simulink model "sim_three_hop"  (R2020b)
settings: Solver=VariableStepAuto  StartTime=0.0  StopTime=1000  RelTol=1e-3  EnableMultiTasking=on
values from neighbouring files (symbols this model uses):
  sim_vars = [ 0, 0.9                8, 1,               8, 1,               8, 1,               inf, inf, inf                rand(1,1)*100000 ]    [main.m]
undefined symbols (not defined in the file or in its folder): m, n
settings Model: SimulationMode=accelerator  Creator=The MathWorks, Inc.  LastModifiedBy=ssmos
settings DataIOCC: LimitDataPoints=on  SaveOperatingPoint=on  SaveFormat=StructureWithTime
settings OptimizationCC: LifeSpan=inf
settings DebuggingCC: AllowSymbolicDim=off  SFUnexpectedBacktrackingDiag=warning  SFNoUnconditionalDefaultTransitionDiag=warning  SFExecutionAtInitializationDiag=none  ArithmeticOperatorsInVariantConditions=warning
settings ModelReferenceCC: PropagateSignalLabelsOutOfModel=off
settings SFSimCC: SimUseLocalCustomCode=off  CustomCodeUndefinedFunction=UseInterfaceOnly
settings RTWCC: RTWUseLocalCustomCode=off
settings CodeAppCC: StateflowObjectComments=on
settings GRTTargetCC: TargetLangStandard=C89/C90 (ANSI)
settings ConfigComp: CovMetricSettings=dw  CovSaveCumulativeToWorkspaceVar=on  CovSaveSingleToWorkspaceVar=on  CovExternalEMLEnable=off  CovSFcnEnable=off

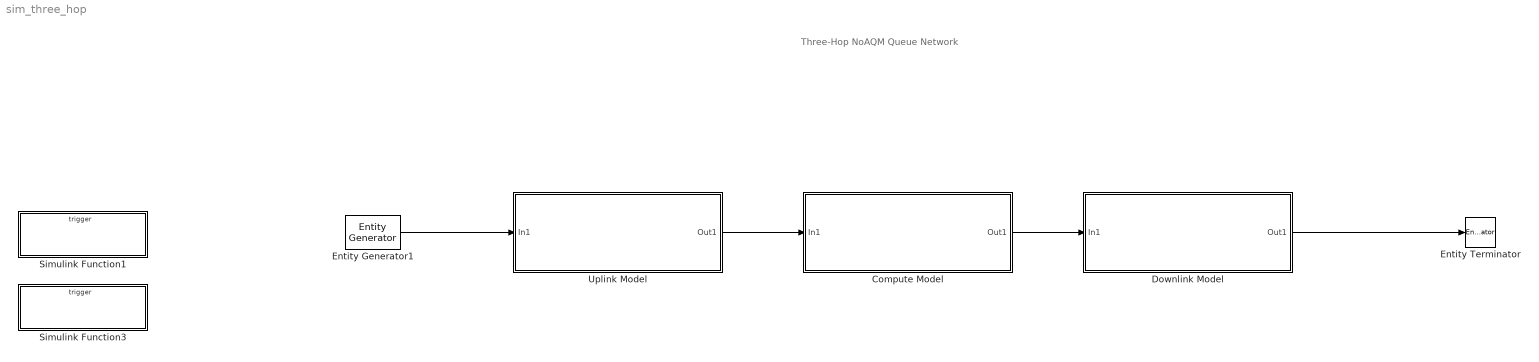
== system sim_three_hop ==
  note: Three-Hop NoAQM Queue Network
  Compute Model : Subsystem
  Downlink Model : Subsystem
  Entity Generator1 : EntityGenerator  OutputPortMessageModes=m  TimeSource=MATLAB action  IntergenerationTimeAction=dt = getArrivalTime(sim_vars(1),sim_vars(2),sim_vars(12));  GenerateAction=|  AttributeName=starttime|queuen_uplink_bu|servern_uplink_bu|queuen_compute_bu|servern_compute_bu|queuen_downlink_bu|servern_downlink_bu|queuen_compute_bc|servern_compute_bc|queuen_downlink_bc|servern_downlink_bc|queuen_downlink_bd|servern_downlink_bd|queuetime_uplink|servicetime_uplink|queuetime_compute|servicetime_compute|queuetime_downlink|servicetime_downlink|endtime  AttributeInitialValue=inf|-1|-1|-1|-1|-1|-1|-1|-1|-1|-1|-1|-1|inf|inf|inf|inf|inf|inf|inf  EntityType=Structured  EntityTypeName=Entity
      | entity.starttime = getCurrentTime();
      | 
      | entity.queuen_uplink_bu = getQueueNUplink();
      | entity.servern_uplink_bu = getServerNUplink();
      | 
      | entity.queuen_compute_bu = getQueueNCompute();
      | entity.servern_compute_bu = getServerNCompute();
      | 
      | entity.queuen_downlink_bu = getQueueNDownlink();
      | entity.servern_downlink_bu = getServerNDownlink();
      | 
      | %[nd,ne,np] = saveCrossNUplink();
      | %entity.crossn_uplink = nd-ne-np;
  Entity Terminator : EntityTerminator  InputPortMessageModes=m  EntryAction=|
      | entity.endtime = getCurrentTime();
      | 
      | saveAttributes([entity.starttime;               ...
      |                 entity.queuen_uplink_bu;        ...
      |                 entity.servern_uplink_bu;       ...
      |                 entity.queuen_compute_bu;       ...
      |                 entity.servern_compute_bu;      ...
      |                 entity.queuen_downlink_bu;      ...
      |                 entity.servern_downlink_bu;     ...
      |                 entity.queuen_compute_bc;       ...
      |                 entity.servern_compute_bc;      ...
      |                 entity.queuen_downlink_bc;      ...
      |                 entity.servern_downlink_bc;     ...
      |                 entity.queuen_downlink_bd;      ...
      |                 entity.servern_downlink_bd;     ...
      |                 entity.queuetime_uplink;        ...
      |                 entity.servicetime_uplink;      ...
      |                 entity.queuetime_compute;       ...
      |                 entity.servicetime_compute;     ...
      |                 entity.queuetime_downlink;      ...
      |                 entity.servicetime_downlink;    ...
      |                 entity.endtime;                 ...
      |                 entitySys.id]);
  Simulink Function1 : Subsystem  TreatAsAtomicUnit=on
  Simulink Function3 : Subsystem  TreatAsAtomicUnit=on
  Uplink Model : Subsystem
  wires:
  Entity Generator1/1 -> Uplink Model/1(In1)
  Uplink Model/1(Out1) -> Compute Model/1(In1)
  Downlink Model/1(Out1) -> Entity Terminator/1
  Compute Model/1(Out1) -> Downlink Model/1(In1)

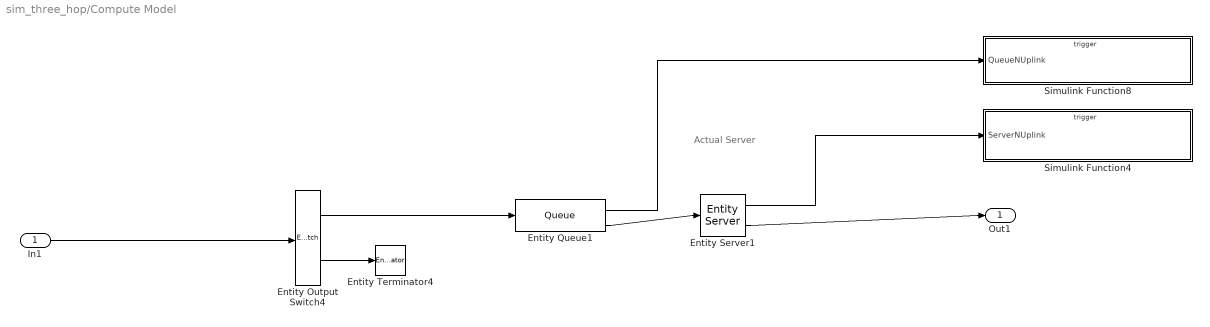
== system sim_three_hop/Compute Model ==
  note: Actual Server
  In1 : Inport
  Entity Output Switch4 : EntityOutputSwitch  InputPortMessageModes=m  OutputPortMessageModes=m,m  SwitchAttributeName=drop_at_source
  Entity Queue1 : Queue  InputPortMessageModes=m  OutputPortMessageModes=n,m  Capacity=sim_vars(10)  NumberEntitiesInBlock=on
      settings: OutputPortMap=o1,o5
  Entity Server1 : EntityServer  InputPortMessageModes=m  OutputPortMessageModes=n,m  Capacity=1  ServiceTimeSource=MATLAB action  ServiceTimeAction=dt = getServiceTimeCompute(sim_vars(5),sim_vars(6),sim_vars(12));  EntryAction=|  ServiceCompleteAction=|  NumberEntitiesInBlock=on
      EntryAction=|
      | % record packet's queue timestamp
      | entity.queuetime_compute = getCurrentTime();
      ServiceCompleteAction=|
      | % record service timestamp
      | entity.servicetime_compute = getCurrentTime();
      | 
      | % record network state in front
      | entity.queuen_downlink_bd = getQueueNDownlink();
      | entity.servern_downlink_bd = getServerNDownlink();
      settings: OutputPortMap=o1,o9
  Entity Terminator4 : EntityTerminator  InputPortMessageModes=m  EntryAction=|
      | saveAttributes([entity.starttime;               ...
      |                 entity.queuen_uplink_bu;        ...
      |                 entity.servern_uplink_bu;       ...
      |                 entity.queuen_compute_bu;       ...
      |                 entity.servern_compute_bu;      ...
      |                 entity.queuen_downlink_bu;      ...
      |                 entity.servern_downlink_bu;     ...
      |                 entity.queuen_compute_bc;       ...
      |                 entity.servern_compute_bc;      ...
      |                 entity.queuen_downlink_bc;      ...
      |                 entity.servern_downlink_bc;     ...
      |                 entity.queuen_downlink_bd;      ...
      |                 entity.servern_downlink_bd;     ...
      |                 entity.queuetime_uplink;        ...
      |                 entity.servicetime_uplink;      ...
      |                 entity.queuetime_compute;       ...
      |                 entity.servicetime_compute;     ...
      |                 entity.queuetime_downlink;      ...
      |                 entity.servicetime_downlink;    ...
      |                 entity.endtime;                 ...
      |                 entitySys.id]);
  Simulink Function4 : Subsystem  TreatAsAtomicUnit=on
  Simulink Function8 : Subsystem  TreatAsAtomicUnit=on
  Out1 : Outport
  wires:
  Entity Queue1/1 -> Simulink Function8/1(QueueNUplink)
  Entity Server1/1 -> Simulink Function4/1(ServerNUplink)
  In1/1 -> Entity Output Switch4/1
  Entity Output Switch4/1 -> Entity Queue1/1
  Entity Queue1/2 -> Entity Server1/1
  Entity Server1/2 -> Out1/1
  Entity Output Switch4/2 -> Entity Terminator4/1

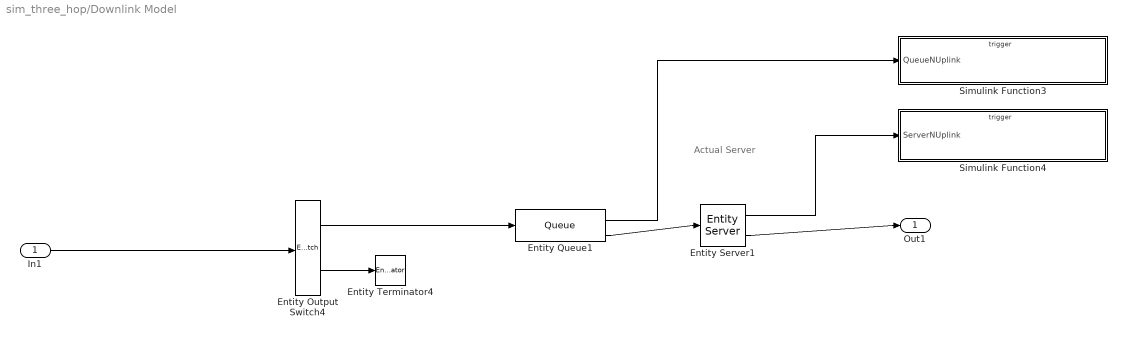
== system sim_three_hop/Downlink Model ==
  note: Actual Server
  In1 : Inport
  Entity Output Switch4 : EntityOutputSwitch  InputPortMessageModes=m  OutputPortMessageModes=m,m  SwitchAttributeName=drop_at_source
  Entity Queue1 : Queue  InputPortMessageModes=m  OutputPortMessageModes=n,m  Capacity=sim_vars(11)  NumberEntitiesInBlock=on
      settings: OutputPortMap=o1,o5
  Entity Server1 : EntityServer  InputPortMessageModes=m  OutputPortMessageModes=n,m  Capacity=1  ServiceTimeSource=MATLAB action  ServiceTimeAction=dt = getServiceTimeDownlink(sim_vars(7),sim_vars(8),sim_vars(12));  EntryAction=|  ServiceCompleteAction=|  NumberEntitiesInBlock=on
      EntryAction=|
      | % record packet's queue timestamp
      | entity.queuetime_downlink = getCurrentTime();
      ServiceCompleteAction=|
      | % record service timestamp
      | entity.servicetime_downlink = getCurrentTime();
      settings: OutputPortMap=o1,o9
  Entity Terminator4 : EntityTerminator  InputPortMessageModes=m  EntryAction=|
      | saveAttributes([entity.starttime;               ...
      |                 entity.queuen_uplink_bu;        ...
      |                 entity.servern_uplink_bu;       ...
      |                 entity.queuen_compute_bu;       ...
      |                 entity.servern_compute_bu;      ...
      |                 entity.queuen_downlink_bu;      ...
      |                 entity.servern_downlink_bu;     ...
      |                 entity.queuen_compute_bc;       ...
      |                 entity.servern_compute_bc;      ...
      |                 entity.queuen_downlink_bc;      ...
      |                 entity.servern_downlink_bc;     ...
      |                 entity.queuen_downlink_bd;      ...
      |                 entity.servern_downlink_bd;     ...
      |                 entity.queuetime_uplink;        ...
      |                 entity.servicetime_uplink;      ...
      |                 entity.queuetime_compute;       ...
      |                 entity.servicetime_compute;     ...
      |                 entity.queuetime_downlink;      ...
      |                 entity.servicetime_downlink;    ...
      |                 entity.endtime;                 ...
      |                 entitySys.id]);
  Simulink Function3 : Subsystem  TreatAsAtomicUnit=on
  Simulink Function4 : Subsystem  TreatAsAtomicUnit=on
  Out1 : Outport
  wires:
  Entity Queue1/1 -> Simulink Function3/1(QueueNUplink)
  Entity Server1/1 -> Simulink Function4/1(ServerNUplink)
  Entity Output Switch4/1 -> Entity Queue1/1
  Entity Queue1/2 -> Entity Server1/1
  Entity Server1/2 -> Out1/1
  Entity Output Switch4/2 -> Entity Terminator4/1
  In1/1 -> Entity Output Switch4/1

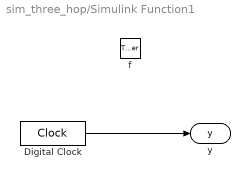
== system sim_three_hop/Simulink Function1 ==
  f : TriggerPort  TriggerType=function-call  IsSimulinkFunction=on  FunctionName=getCurrentTime  VariantControl=(inherit)
  Digital Clock : DigitalClock  SampleTime=-1
  y : ArgOut  DisableCoverage=on  ArgumentName=y
  wires:
  Digital Clock/1 -> y/1

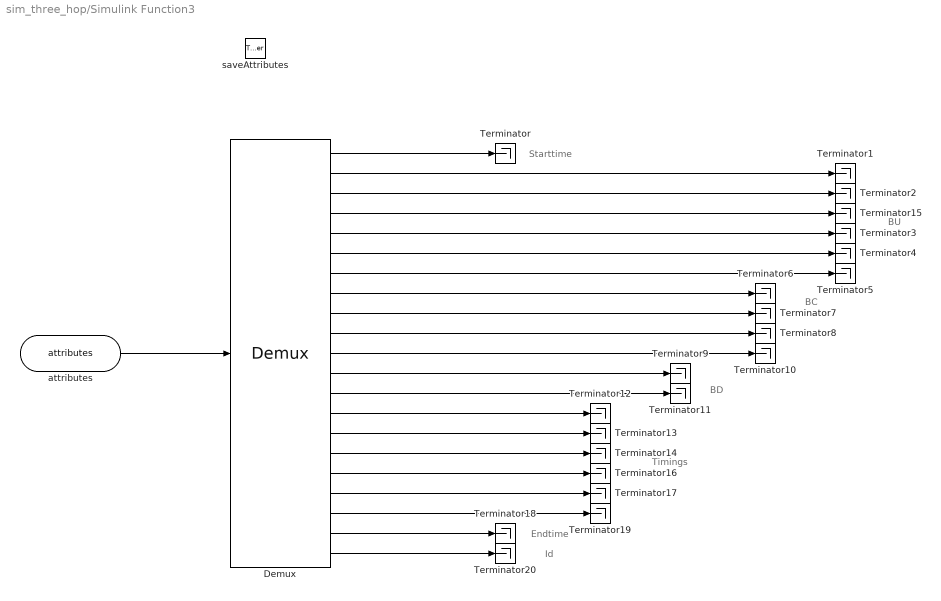
== system sim_three_hop/Simulink Function3 ==
  note: Id
  note: Endtime
  note: Starttime
  note: Timings
  note: BU
  note: BC
  note: BD
  saveAttributes : TriggerPort  TriggerType=function-call  IsSimulinkFunction=on  FunctionName=saveAttributes  VariantControl=(inherit)
  Demux : Demux  Outputs=21
      settings: DisplayOption=none
  Terminator{,1..20} (21 alike) : Terminator
  attributes : ArgIn  DisableCoverage=on  PortDimensions=21  ArgumentName=attributes
  wires:
  attributes/1 -> Demux/1
  Demux/1 -> Terminator/1
  Demux/2 -> Terminator1/1
  Demux/3 -> Terminator2/1
  Demux/7 -> Terminator5/1
  Demux/5 -> Terminator3/1
  Demux/6 -> Terminator4/1
  Demux/8 -> Terminator6/1
  Demux/4 -> Terminator15/1
  Demux/9 -> Terminator7/1
  Demux/10 -> Terminator8/1
  Demux/11 -> Terminator10/1
  Demux/12 -> Terminator9/1
  Demux/13 -> Terminator11/1
  Demux/14 -> Terminator12/1
  Demux/15 -> Terminator13/1
  Demux/16 -> Terminator14/1
  Demux/17 -> Terminator16/1
  Demux/18 -> Terminator17/1
  Demux/19 -> Terminator19/1
  Demux/20 -> Terminator18/1
  Demux/21 -> Terminator20/1

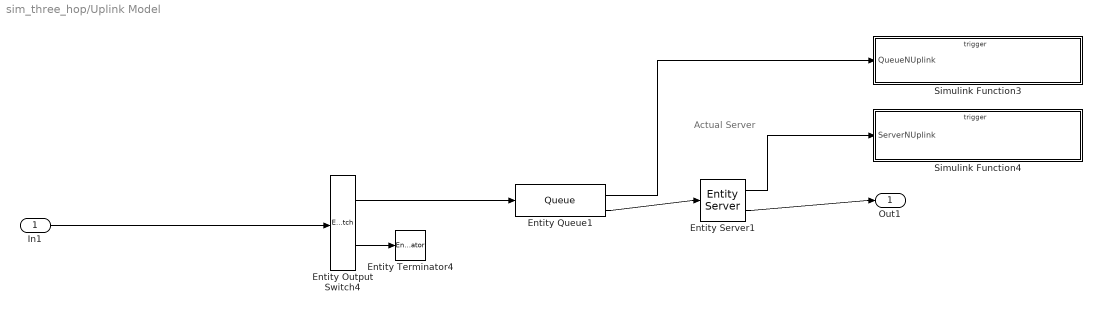
== system sim_three_hop/Uplink Model ==
  note: Actual Server
  In1 : Inport
  Entity Output Switch4 : EntityOutputSwitch  InputPortMessageModes=m  OutputPortMessageModes=m,m  SwitchAttributeName=drop_at_source
  Entity Queue1 : Queue  InputPortMessageModes=m  OutputPortMessageModes=n,m  Capacity=sim_vars(9)  NumberEntitiesInBlock=on
      settings: OutputPortMap=o1,o5
  Entity Server1 : EntityServer  InputPortMessageModes=m  OutputPortMessageModes=n,m  Capacity=1  ServiceTimeSource=MATLAB action  ServiceTimeAction=dt = getServiceTimeUplink(sim_vars(3),sim_vars(4),sim_vars(12));  EntryAction=|  ServiceCompleteAction=|  NumberEntitiesInBlock=on
      EntryAction=|
      | % update packet's queue timestamp
      | entity.queuetime_uplink = getCurrentTime();
      ServiceCompleteAction=|
      | % update service time
      | entity.servicetime_uplink = getCurrentTime();
      | 
      | % save network state in front
      | entity.queuen_compute_bc = getQueueNCompute();
      | entity.servern_compute_bc = getServerNCompute();
      | 
      | entity.queuen_downlink_bc = getQueueNDownlink();
      | entity.servern_downlink_bc = getServerNDownlink();
      settings: OutputPortMap=o1,o9
  Entity Terminator4 : EntityTerminator  InputPortMessageModes=m  EntryAction=|
      | saveAttributes([entity.starttime;               ...
      |                 entity.queuen_uplink_bu;        ...
      |                 entity.servern_uplink_bu;       ...
      |                 entity.queuen_compute_bu;       ...
      |                 entity.servern_compute_bu;      ...
      |                 entity.queuen_downlink_bu;      ...
      |                 entity.servern_downlink_bu;     ...
      |                 entity.queuen_compute_bc;       ...
      |                 entity.servern_compute_bc;      ...
      |                 entity.queuen_downlink_bc;      ...
      |                 entity.servern_downlink_bc;     ...
      |                 entity.queuen_downlink_bd;      ...
      |                 entity.servern_downlink_bd;     ...
      |                 entity.queuetime_uplink;        ...
      |                 entity.servicetime_uplink;      ...
      |                 entity.queuetime_compute;       ...
      |                 entity.servicetime_compute;     ...
      |                 entity.queuetime_downlink;      ...
      |                 entity.servicetime_downlink;    ...
      |                 entity.endtime;                 ...
      |                 entitySys.id]);
  Simulink Function3 : Subsystem  TreatAsAtomicUnit=on
  Simulink Function4 : Subsystem  TreatAsAtomicUnit=on
  Out1 : Outport
  wires:
  Entity Queue1/1 -> Simulink Function3/1(QueueNUplink)
  Entity Server1/1 -> Simulink Function4/1(ServerNUplink)
  In1/1 -> Entity Output Switch4/1
  Entity Output Switch4/1 -> Entity Queue1/1
  Entity Queue1/2 -> Entity Server1/1
  Entity Server1/2 -> Out1/1
  Entity Output Switch4/2 -> Entity Terminator4/1

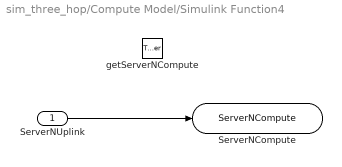
== system sim_three_hop/Compute Model/Simulink Function4 ==
  ServerNUplink : Inport
  getServerNCompute : TriggerPort  TriggerType=function-call  IsSimulinkFunction=on  FunctionName=getServerNCompute  VariantControl=(inherit)
  ServerNCompute : ArgOut  DisableCoverage=on  ArgumentName=ServerNCompute
  wires:
  ServerNUplink/1 -> ServerNCompute/1

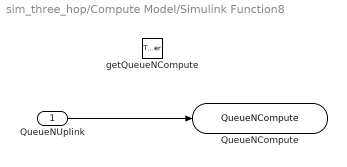
== system sim_three_hop/Compute Model/Simulink Function8 ==
  QueueNUplink : Inport
  getQueueNCompute : TriggerPort  TriggerType=function-call  IsSimulinkFunction=on  FunctionName=getQueueNCompute  VariantControl=(inherit)
  QueueNCompute : ArgOut  DisableCoverage=on  ArgumentName=QueueNCompute
  wires:
  QueueNUplink/1 -> QueueNCompute/1

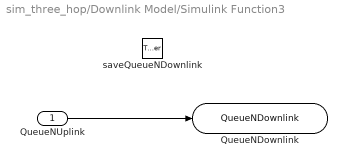
== system sim_three_hop/Downlink Model/Simulink Function3 ==
  QueueNUplink : Inport
  saveQueueNDownlink : TriggerPort  TriggerType=function-call  IsSimulinkFunction=on  FunctionName=getQueueNDownlink  VariantControl=(inherit)
  QueueNDownlink : ArgOut  DisableCoverage=on  ArgumentName=QueueNDownlink
  wires:
  QueueNUplink/1 -> QueueNDownlink/1

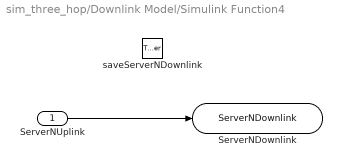
== system sim_three_hop/Downlink Model/Simulink Function4 ==
  ServerNUplink : Inport
  saveServerNDownlink : TriggerPort  TriggerType=function-call  IsSimulinkFunction=on  FunctionName=getServerNDownlink  VariantControl=(inherit)
  ServerNDownlink : ArgOut  DisableCoverage=on  ArgumentName=ServerNDownlink
  wires:
  ServerNUplink/1 -> ServerNDownlink/1

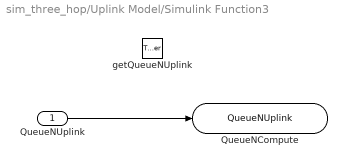
== system sim_three_hop/Uplink Model/Simulink Function3 ==
  QueueNUplink : Inport
  getQueueNUplink : TriggerPort  TriggerType=function-call  IsSimulinkFunction=on  FunctionName=getQueueNUplink  VariantControl=(inherit)
  QueueNCompute : ArgOut  DisableCoverage=on  ArgumentName=QueueNUplink
  wires:
  QueueNUplink/1 -> QueueNCompute/1

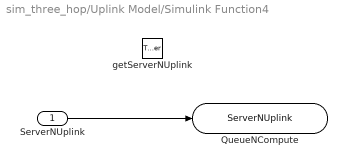
== system sim_three_hop/Uplink Model/Simulink Function4 ==
  ServerNUplink : Inport
  getServerNUplink : TriggerPort  TriggerType=function-call  IsSimulinkFunction=on  FunctionName=getServerNUplink  VariantControl=(inherit)
  QueueNCompute : ArgOut  DisableCoverage=on  ArgumentName=ServerNUplink
  wires:
  ServerNUplink/1 -> QueueNCompute/1
